simulink library "Lib_JARVISPH2_deVCU_Anlg"  (R2019b)
settings: Solver=ode45  StartTime=0.0  StopTime=10.0  RelTol=1e-3  EnableMultiTasking=on
settings Model: Creator=kmansour  LastModifiedBy=User
settings DataIOCC: LimitDataPoints=on  SaveFormat=Array  ReturnWorkspaceOutputs=off
settings OptimizationCC: LifeSpan=inf
settings DebuggingCC: AllowSymbolicDim=off  SFUnexpectedBacktrackingDiag=warning  SFNoUnconditionalDefaultTransitionDiag=warning  SFExecutionAtInitializationDiag=none  ArithmeticOperatorsInVariantConditions=warning
settings HardwareCC: ProdBitPerPointer=32  ProdBitPerSizeT=32  ProdBitPerPtrDiffT=32  ProdLargestAtomicFloat=None  ProdIntDivRoundTo=Undefined  ProdEndianess=Unspecified  ProdWordSize=32  ProdHWDeviceType=32-bit Generic
settings ModelReferenceCC: PropagateSignalLabelsOutOfModel=off
settings SFSimCC: SimUseLocalCustomCode=off  CustomCodeUndefinedFunction=UseInterfaceOnly
settings RTWCC: RTWUseLocalCustomCode=off
settings CodeAppCC: StateflowObjectComments=on
settings GRTTargetCC: TargetLangStandard=C89/C90 (ANSI)  GeneratePreprocessorConditionals=Disable all
settings ConfigComp: CovMetricSettings=dw  CovHtmlReporting=on  CovSaveCumulativeToWorkspaceVar=on  CovSaveSingleToWorkspaceVar=on  CovExternalEMLEnable=off

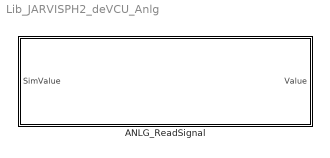
== system Lib_JARVISPH2_deVCU_Anlg ==
  ANLG_ReadSignal : Subsystem  TreatAsAtomicUnit=on  mask{PARAM_ID=ECU_ANLG_ECU_AC_PP_SIG}
      mask prompts: PARAM_ID "Choose a Signal"
      mask TypeOptions PARAM_ID: ECU_ANLG_ECU_AC_PP_SIG | ECU_ANLG_VCU_AUX24V_P49 | ECU_ANLG_NONAME_PIN_P60 | ECU_ANLG_BCS_TEMP2_SENSOR_P65 | ECU_ANLG_TCS_TEMP_SENSORINLET_P67 | ECU_ANLG_TCS_TEMP_SENSOROUTLET_P68 | ECU_ANLG_TCS_TEMP_SENSORINLET_P69 | ECU_ANLG_ECU_VOLTAGE
      mask Display:
      | image(imread('devcu_final.png'),'top-left');
      | color('black');
      | port_label('input', 1, 'SimValue');
      | port_label('output', 1, 'Value');
      | 
      | strCell =get_param(gcb, 'MaskValues');
      | strCell = strtrim(strCell);
      | str = strCell{1};
      | str = strrep(str, '_', '\_');
      | disp(str, 'texmode', 'on');

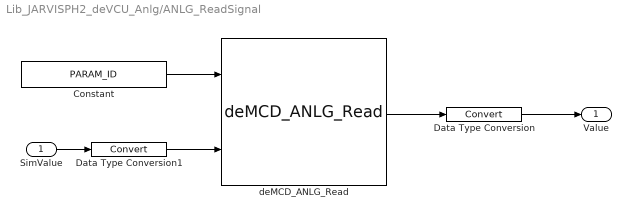
== system Lib_JARVISPH2_deVCU_Anlg/ANLG_ReadSignal ==
  SimValue : Inport
  Constant : Constant  Value=PARAM_ID
  Data Type Conversion : DataTypeConversion
  Data Type Conversion1 : DataTypeConversion
  deMCD_ANLG_Read : S-Function  FunctionName=deMCD_ANLG_Read  SFunctionDeploymentMode=off  EnableBusSupport=off
      mask Display:
      | image(imread('logo_deMCD_white_background.png'),'center');
      | color('black');
      | port_label('input', 1, 'ID');
      | port_label('input', 2, 'SimValue');
      | port_label('output', 1, 'Value');
  Value : Outport
  wires:
  deMCD_ANLG_Read/1 -> Data Type Conversion/1
  Constant/1 -> deMCD_ANLG_Read/1
  Data Type Conversion/1 -> Value/1
  Data Type Conversion1/1 -> deMCD_ANLG_Read/2
  SimValue/1 -> Data Type Conversion1/1
